simulink model "SYSTEMCOMPLEX"  (R2025b)
settings: Solver=VariableStepAuto  StartTime=0.0  StopTime=10.0  RelTol=1e-3
(part 2 of 2)

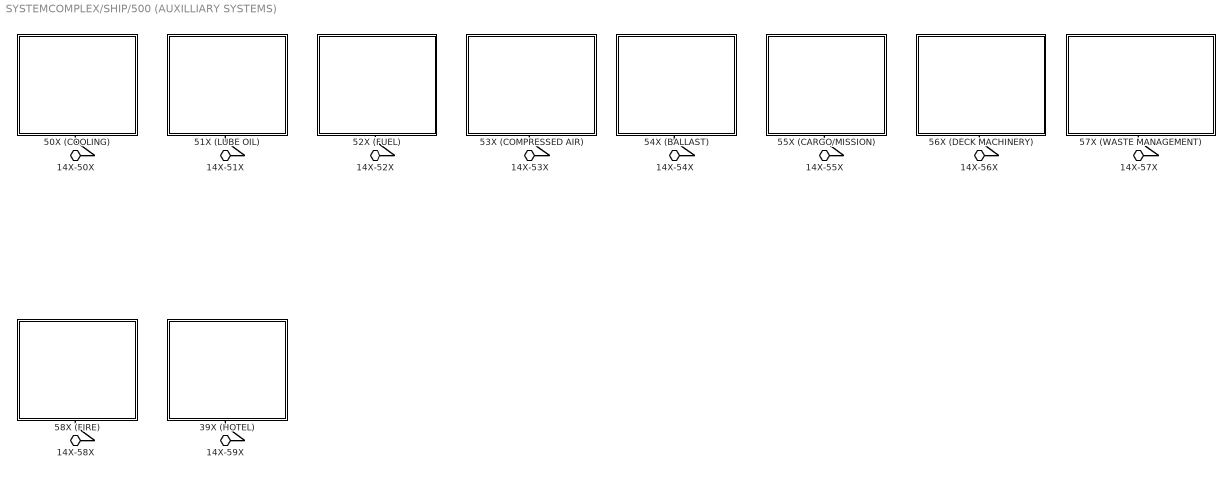
== system SYSTEMCOMPLEX/SHIP/500 (AUXILLIARY SYSTEMS) ==
  39X (HOTEL) : Subsystem
      settings: PortSchema="{\"entries\":[{\"content\":{\"headerSize\":26,\"margin\":15,\"minimumSpacing\":25,\"sides\":[{\"content\":{},\"type\":\"ConnectorPlacement.EquallySpacedRectSide\",\"uuid\":\"c62bca68-e99b-4d4a-8c3b-c9a3c6520291\"},{\"content\":{\"side\":\"RIGHT\"},\"type\":\"ConnectorPlacement.EquallySpacedRectSide\",\"uuid\":\"9f78cd75-5645-4950-8d66-9f0d33627f1f\"},{\"content\":{\"side\":\"TOP\"},\"type\":\"ConnectorPlacement.EquallySpacedRectSide\",\"uuid\":\"f95077c9-4a6b-4bf1-8b13-59697d659817\"},{\"content\":{\"connectorIds\":[\"RConn1\"],\"side\":\"BOTTOM\"},\"type\":\"ConnectorPlacement.EquallySpacedRectSide\",\"uuid\":\"0006d70a-f92f-457d-a614-8f3c10052d85\"}]},\"type\":\"ConnectorPlacement.EquallySpacedConnector\",\"uuid\":\"da1ef182-4ed3-4fb4-823f-e8eb0a5ecd15\"}],\"packageUris\":[\"http://schema.mathworks.com/mf0/Connector/R2020b\"],\"version\":\"1.0\"}"
  50X (COOLING) : Subsystem
      settings: PortSchema="{\"entries\":[{\"content\":{\"headerSize\":26,\"margin\":15,\"minimumSpacing\":25,\"sides\":[{\"content\":{},\"type\":\"ConnectorPlacement.EquallySpacedRectSide\",\"uuid\":\"c62bca68-e99b-4d4a-8c3b-c9a3c6520291\"},{\"content\":{\"side\":\"RIGHT\"},\"type\":\"ConnectorPlacement.EquallySpacedRectSide\",\"uuid\":\"9f78cd75-5645-4950-8d66-9f0d33627f1f\"},{\"content\":{\"side\":\"TOP\"},\"type\":\"ConnectorPlacement.EquallySpacedRectSide\",\"uuid\":\"f95077c9-4a6b-4bf1-8b13-59697d659817\"},{\"content\":{\"connectorIds\":[\"RConn1\"],\"side\":\"BOTTOM\"},\"type\":\"ConnectorPlacement.EquallySpacedRectSide\",\"uuid\":\"c6240b2d-810b-4c18-b4a4-281a824149ba\"}]},\"type\":\"ConnectorPlacement.EquallySpacedConnector\",\"uuid\":\"da1ef182-4ed3-4fb4-823f-e8eb0a5ecd15\"}],\"packageUris\":[\"http://schema.mathworks.com/mf0/Connector/R2020b\"],\"version\":\"1.0\"}"
  51X (LUBE OIL) : Subsystem
      settings: PortSchema="{\"entries\":[{\"content\":{\"headerSize\":26,\"margin\":15,\"minimumSpacing\":25,\"sides\":[{\"content\":{},\"type\":\"ConnectorPlacement.EquallySpacedRectSide\",\"uuid\":\"c62bca68-e99b-4d4a-8c3b-c9a3c6520291\"},{\"content\":{\"side\":\"RIGHT\"},\"type\":\"ConnectorPlacement.EquallySpacedRectSide\",\"uuid\":\"9f78cd75-5645-4950-8d66-9f0d33627f1f\"},{\"content\":{\"side\":\"TOP\"},\"type\":\"ConnectorPlacement.EquallySpacedRectSide\",\"uuid\":\"f95077c9-4a6b-4bf1-8b13-59697d659817\"},{\"content\":{\"connectorIds\":[\"RConn1\"],\"side\":\"BOTTOM\"},\"type\":\"ConnectorPlacement.EquallySpacedRectSide\",\"uuid\":\"3fff4ade-ce74-4018-83c1-67b82f153eaa\"}]},\"type\":\"ConnectorPlacement.EquallySpacedConnector\",\"uuid\":\"da1ef182-4ed3-4fb4-823f-e8eb0a5ecd15\"}],\"packageUris\":[\"http://schema.mathworks.com/mf0/Connector/R2020b\"],\"version\":\"1.0\"}"
  52X (FUEL) : Subsystem
      settings: PortSchema="{\"entries\":[{\"content\":{\"headerSize\":26,\"margin\":15,\"minimumSpacing\":25,\"sides\":[{\"content\":{},\"type\":\"ConnectorPlacement.EquallySpacedRectSide\",\"uuid\":\"c62bca68-e99b-4d4a-8c3b-c9a3c6520291\"},{\"content\":{\"side\":\"RIGHT\"},\"type\":\"ConnectorPlacement.EquallySpacedRectSide\",\"uuid\":\"9f78cd75-5645-4950-8d66-9f0d33627f1f\"},{\"content\":{\"side\":\"TOP\"},\"type\":\"ConnectorPlacement.EquallySpacedRectSide\",\"uuid\":\"f95077c9-4a6b-4bf1-8b13-59697d659817\"},{\"content\":{\"connectorIds\":[\"RConn1\"],\"side\":\"BOTTOM\"},\"type\":\"ConnectorPlacement.EquallySpacedRectSide\",\"uuid\":\"83459f23-a1ce-4fbc-97a5-e0f72e97561e\"}]},\"type\":\"ConnectorPlacement.EquallySpacedConnector\",\"uuid\":\"da1ef182-4ed3-4fb4-823f-e8eb0a5ecd15\"}],\"packageUris\":[\"http://schema.mathworks.com/mf0/Connector/R2020b\"],\"version\":\"1.0\"}"
  53X (COMPRESSED AIR) : Subsystem
      settings: PortSchema="{\"entries\":[{\"content\":{\"headerSize\":26,\"margin\":15,\"minimumSpacing\":25,\"sides\":[{\"content\":{},\"type\":\"ConnectorPlacement.EquallySpacedRectSide\",\"uuid\":\"c62bca68-e99b-4d4a-8c3b-c9a3c6520291\"},{\"content\":{\"side\":\"RIGHT\"},\"type\":\"ConnectorPlacement.EquallySpacedRectSide\",\"uuid\":\"9f78cd75-5645-4950-8d66-9f0d33627f1f\"},{\"content\":{\"side\":\"TOP\"},\"type\":\"ConnectorPlacement.EquallySpacedRectSide\",\"uuid\":\"f95077c9-4a6b-4bf1-8b13-59697d659817\"},{\"content\":{\"connectorIds\":[\"RConn1\"],\"side\":\"BOTTOM\"},\"type\":\"ConnectorPlacement.EquallySpacedRectSide\",\"uuid\":\"74713995-6afe-49df-9f00-ac1603891ac3\"}]},\"type\":\"ConnectorPlacement.EquallySpacedConnector\",\"uuid\":\"da1ef182-4ed3-4fb4-823f-e8eb0a5ecd15\"}],\"packageUris\":[\"http://schema.mathworks.com/mf0/Connector/R2020b\"],\"version\":\"1.0\"}"
  54X (BALLAST) : Subsystem
      settings: PortSchema="{\"entries\":[{\"content\":{\"headerSize\":26,\"margin\":15,\"minimumSpacing\":25,\"sides\":[{\"content\":{},\"type\":\"ConnectorPlacement.EquallySpacedRectSide\",\"uuid\":\"c62bca68-e99b-4d4a-8c3b-c9a3c6520291\"},{\"content\":{\"side\":\"RIGHT\"},\"type\":\"ConnectorPlacement.EquallySpacedRectSide\",\"uuid\":\"9f78cd75-5645-4950-8d66-9f0d33627f1f\"},{\"content\":{\"side\":\"TOP\"},\"type\":\"ConnectorPlacement.EquallySpacedRectSide\",\"uuid\":\"f95077c9-4a6b-4bf1-8b13-59697d659817\"},{\"content\":{\"connectorIds\":[\"RConn1\"],\"side\":\"BOTTOM\"},\"type\":\"ConnectorPlacement.EquallySpacedRectSide\",\"uuid\":\"68d91af7-5bf5-42be-a1d8-d4884acaee75\"}]},\"type\":\"ConnectorPlacement.EquallySpacedConnector\",\"uuid\":\"da1ef182-4ed3-4fb4-823f-e8eb0a5ecd15\"}],\"packageUris\":[\"http://schema.mathworks.com/mf0/Connector/R2020b\"],\"version\":\"1.0\"}"
  55X (CARGO/MISSION) : Subsystem
      settings: PortSchema="{\"entries\":[{\"content\":{\"headerSize\":26,\"margin\":15,\"minimumSpacing\":25,\"sides\":[{\"content\":{},\"type\":\"ConnectorPlacement.EquallySpacedRectSide\",\"uuid\":\"c62bca68-e99b-4d4a-8c3b-c9a3c6520291\"},{\"content\":{\"side\":\"RIGHT\"},\"type\":\"ConnectorPlacement.EquallySpacedRectSide\",\"uuid\":\"9f78cd75-5645-4950-8d66-9f0d33627f1f\"},{\"content\":{\"side\":\"TOP\"},\"type\":\"ConnectorPlacement.EquallySpacedRectSide\",\"uuid\":\"f95077c9-4a6b-4bf1-8b13-59697d659817\"},{\"content\":{\"connectorIds\":[\"RConn1\"],\"side\":\"BOTTOM\"},\"type\":\"ConnectorPlacement.EquallySpacedRectSide\",\"uuid\":\"082ae5ab-4f38-4cbc-8d3b-78d157006bcc\"}]},\"type\":\"ConnectorPlacement.EquallySpacedConnector\",\"uuid\":\"da1ef182-4ed3-4fb4-823f-e8eb0a5ecd15\"}],\"packageUris\":[\"http://schema.mathworks.com/mf0/Connector/R2020b\"],\"version\":\"1.0\"}"
  56X (DECK MACHINERY) : Subsystem
      settings: PortSchema="{\"entries\":[{\"content\":{\"headerSize\":26,\"margin\":15,\"minimumSpacing\":25,\"sides\":[{\"content\":{},\"type\":\"ConnectorPlacement.EquallySpacedRectSide\",\"uuid\":\"c62bca68-e99b-4d4a-8c3b-c9a3c6520291\"},{\"content\":{\"side\":\"RIGHT\"},\"type\":\"ConnectorPlacement.EquallySpacedRectSide\",\"uuid\":\"9f78cd75-5645-4950-8d66-9f0d33627f1f\"},{\"content\":{\"side\":\"TOP\"},\"type\":\"ConnectorPlacement.EquallySpacedRectSide\",\"uuid\":\"f95077c9-4a6b-4bf1-8b13-59697d659817\"},{\"content\":{\"connectorIds\":[\"RConn1\"],\"side\":\"BOTTOM\"},\"type\":\"ConnectorPlacement.EquallySpacedRectSide\",\"uuid\":\"aa3da118-94c8-43a4-9a24-28ea9b935bf4\"}]},\"type\":\"ConnectorPlacement.EquallySpacedConnector\",\"uuid\":\"da1ef182-4ed3-4fb4-823f-e8eb0a5ecd15\"}],\"packageUris\":[\"http://schema.mathworks.com/mf0/Connector/R2020b\"],\"version\":\"1.0\"}"
  57X (WASTE MANAGEMENT) : Subsystem
      settings: PortSchema="{\"entries\":[{\"content\":{\"headerSize\":26,\"margin\":15,\"minimumSpacing\":25,\"sides\":[{\"content\":{},\"type\":\"ConnectorPlacement.EquallySpacedRectSide\",\"uuid\":\"c62bca68-e99b-4d4a-8c3b-c9a3c6520291\"},{\"content\":{\"side\":\"RIGHT\"},\"type\":\"ConnectorPlacement.EquallySpacedRectSide\",\"uuid\":\"9f78cd75-5645-4950-8d66-9f0d33627f1f\"},{\"content\":{\"side\":\"TOP\"},\"type\":\"ConnectorPlacement.EquallySpacedRectSide\",\"uuid\":\"f95077c9-4a6b-4bf1-8b13-59697d659817\"},{\"content\":{\"connectorIds\":[\"RConn1\"],\"side\":\"BOTTOM\"},\"type\":\"ConnectorPlacement.EquallySpacedRectSide\",\"uuid\":\"a20644fe-ab63-4955-9ccf-f975c8687a67\"}]},\"type\":\"ConnectorPlacement.EquallySpacedConnector\",\"uuid\":\"da1ef182-4ed3-4fb4-823f-e8eb0a5ecd15\"}],\"packageUris\":[\"http://schema.mathworks.com/mf0/Connector/R2020b\"],\"version\":\"1.0\"}"
  58X (FIRE) : Subsystem
      settings: PortSchema="{\"entries\":[{\"content\":{\"headerSize\":26,\"margin\":15,\"minimumSpacing\":25,\"sides\":[{\"content\":{},\"type\":\"ConnectorPlacement.EquallySpacedRectSide\",\"uuid\":\"c62bca68-e99b-4d4a-8c3b-c9a3c6520291\"},{\"content\":{\"side\":\"RIGHT\"},\"type\":\"ConnectorPlacement.EquallySpacedRectSide\",\"uuid\":\"9f78cd75-5645-4950-8d66-9f0d33627f1f\"},{\"content\":{\"side\":\"TOP\"},\"type\":\"ConnectorPlacement.EquallySpacedRectSide\",\"uuid\":\"f95077c9-4a6b-4bf1-8b13-59697d659817\"},{\"content\":{\"connectorIds\":[\"RConn1\"],\"side\":\"BOTTOM\"},\"type\":\"ConnectorPlacement.EquallySpacedRectSide\",\"uuid\":\"000ad661-d3a1-4abe-a6ec-7b31413b8243\"}]},\"type\":\"ConnectorPlacement.EquallySpacedConnector\",\"uuid\":\"da1ef182-4ed3-4fb4-823f-e8eb0a5ecd15\"}],\"packageUris\":[\"http://schema.mathworks.com/mf0/Connector/R2020b\"],\"version\":\"1.0\"}"
  14X-50X : PMIOPort  Side=Left
  14X-51X : PMIOPort  Port=2  Side=Left
  14X-52X : PMIOPort  Port=3  Side=Left
  14X-53X : PMIOPort  Port=4  Side=Left
  14X-54X : PMIOPort  Port=5  Side=Left
  14X-55X : PMIOPort  Port=6  Side=Left
  14X-56X : PMIOPort  Port=7  Side=Left
  14X-57X : PMIOPort  Port=8  Side=Left
  14X-58X : PMIOPort  Port=9  Side=Left
  14X-59X : PMIOPort  Port=10  Side=Left
  connections:
  14X-50X/RConn1 -- 50X (COOLING)/RConn1
  14X-51X/RConn1 -- 51X (LUBE OIL)/RConn1
  14X-52X/RConn1 -- 52X (FUEL)/RConn1
  14X-53X/RConn1 -- 53X (COMPRESSED AIR)/RConn1
  14X-54X/RConn1 -- 54X (BALLAST)/RConn1
  14X-55X/RConn1 -- 55X (CARGO/MISSION)/RConn1
  14X-56X/RConn1 -- 56X (DECK MACHINERY)/RConn1
  14X-57X/RConn1 -- 57X (WASTE MANAGEMENT)/RConn1
  14X-58X/RConn1 -- 58X (FIRE)/RConn1
  14X-59X/RConn1 -- 39X (HOTEL)/RConn1

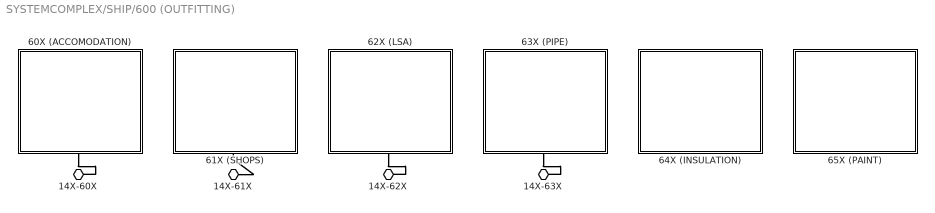
== system SYSTEMCOMPLEX/SHIP/600 (OUTFITTING) ==
  60X (ACCOMODATION) : Subsystem
      settings: PortSchema="{\"entries\":[{\"content\":{\"headerSize\":26,\"margin\":15,\"minimumSpacing\":25,\"sides\":[{\"content\":{},\"type\":\"ConnectorPlacement.EquallySpacedRectSide\",\"uuid\":\"c62bca68-e99b-4d4a-8c3b-c9a3c6520291\"},{\"content\":{\"side\":\"RIGHT\"},\"type\":\"ConnectorPlacement.EquallySpacedRectSide\",\"uuid\":\"9f78cd75-5645-4950-8d66-9f0d33627f1f\"},{\"content\":{\"side\":\"TOP\"},\"type\":\"ConnectorPlacement.EquallySpacedRectSide\",\"uuid\":\"f95077c9-4a6b-4bf1-8b13-59697d659817\"},{\"content\":{\"connectorIds\":[\"RConn1\"],\"side\":\"BOTTOM\"},\"type\":\"ConnectorPlacement.EquallySpacedRectSide\",\"uuid\":\"e1b75886-8c6a-41df-87a3-90c3eee2745e\"}]},\"type\":\"ConnectorPlacement.EquallySpacedConnector\",\"uuid\":\"da1ef182-4ed3-4fb4-823f-e8eb0a5ecd15\"}],\"packageUris\":[\"http://schema.mathworks.com/mf0/Connector/R2020b\"],\"version\":\"1.0\"}"
  61X (SHOPS) : Subsystem
      settings: PortSchema="{\"entries\":[{\"content\":{\"headerSize\":26,\"margin\":15,\"minimumSpacing\":25,\"sides\":[{\"content\":{},\"type\":\"ConnectorPlacement.EquallySpacedRectSide\",\"uuid\":\"c62bca68-e99b-4d4a-8c3b-c9a3c6520291\"},{\"content\":{\"side\":\"RIGHT\"},\"type\":\"ConnectorPlacement.EquallySpacedRectSide\",\"uuid\":\"9f78cd75-5645-4950-8d66-9f0d33627f1f\"},{\"content\":{\"side\":\"TOP\"},\"type\":\"ConnectorPlacement.EquallySpacedRectSide\",\"uuid\":\"f95077c9-4a6b-4bf1-8b13-59697d659817\"},{\"content\":{\"connectorIds\":[\"RConn1\"],\"side\":\"BOTTOM\"},\"type\":\"ConnectorPlacement.EquallySpacedRectSide\",\"uuid\":\"eda74852-aada-4e88-83db-568f63a98b4f\"}]},\"type\":\"ConnectorPlacement.EquallySpacedConnector\",\"uuid\":\"da1ef182-4ed3-4fb4-823f-e8eb0a5ecd15\"}],\"packageUris\":[\"http://schema.mathworks.com/mf0/Connector/R2020b\"],\"version\":\"1.0\"}"
  62X (LSA) : Subsystem
      settings: PortSchema="{\"entries\":[{\"content\":{\"headerSize\":26,\"margin\":15,\"minimumSpacing\":25,\"sides\":[{\"content\":{},\"type\":\"ConnectorPlacement.EquallySpacedRectSide\",\"uuid\":\"c62bca68-e99b-4d4a-8c3b-c9a3c6520291\"},{\"content\":{\"side\":\"RIGHT\"},\"type\":\"ConnectorPlacement.EquallySpacedRectSide\",\"uuid\":\"9f78cd75-5645-4950-8d66-9f0d33627f1f\"},{\"content\":{\"side\":\"TOP\"},\"type\":\"ConnectorPlacement.EquallySpacedRectSide\",\"uuid\":\"f95077c9-4a6b-4bf1-8b13-59697d659817\"},{\"content\":{\"connectorIds\":[\"RConn1\"],\"side\":\"BOTTOM\"},\"type\":\"ConnectorPlacement.EquallySpacedRectSide\",\"uuid\":\"eb68c783-c2b7-425c-a30e-1e7ae8b8046b\"}]},\"type\":\"ConnectorPlacement.EquallySpacedConnector\",\"uuid\":\"da1ef182-4ed3-4fb4-823f-e8eb0a5ecd15\"}],\"packageUris\":[\"http://schema.mathworks.com/mf0/Connector/R2020b\"],\"version\":\"1.0\"}"
  63X (PIPE) : Subsystem
      settings: PortSchema="{\"entries\":[{\"content\":{\"headerSize\":26,\"margin\":15,\"minimumSpacing\":25,\"sides\":[{\"content\":{},\"type\":\"ConnectorPlacement.EquallySpacedRectSide\",\"uuid\":\"c62bca68-e99b-4d4a-8c3b-c9a3c6520291\"},{\"content\":{\"side\":\"RIGHT\"},\"type\":\"ConnectorPlacement.EquallySpacedRectSide\",\"uuid\":\"9f78cd75-5645-4950-8d66-9f0d33627f1f\"},{\"content\":{\"side\":\"TOP\"},\"type\":\"ConnectorPlacement.EquallySpacedRectSide\",\"uuid\":\"f95077c9-4a6b-4bf1-8b13-59697d659817\"},{\"content\":{\"connectorIds\":[\"RConn1\"],\"side\":\"BOTTOM\"},\"type\":\"ConnectorPlacement.EquallySpacedRectSide\",\"uuid\":\"9d615349-c26c-46cb-ae8c-7a410c7bc294\"}]},\"type\":\"ConnectorPlacement.EquallySpacedConnector\",\"uuid\":\"da1ef182-4ed3-4fb4-823f-e8eb0a5ecd15\"}],\"packageUris\":[\"http://schema.mathworks.com/mf0/Connector/R2020b\"],\"version\":\"1.0\"}"
  64X (INSULATION) : Subsystem
      settings: PortSchema="{\"entries\":[{\"content\":{\"headerSize\":26,\"margin\":15,\"minimumSpacing\":25,\"sides\":[{\"content\":{},\"type\":\"ConnectorPlacement.EquallySpacedRectSide\",\"uuid\":\"c62bca68-e99b-4d4a-8c3b-c9a3c6520291\"},{\"content\":{\"side\":\"RIGHT\"},\"type\":\"ConnectorPlacement.EquallySpacedRectSide\",\"uuid\":\"9f78cd75-5645-4950-8d66-9f0d33627f1f\"},{\"content\":{\"side\":\"TOP\"},\"type\":\"ConnectorPlacement.EquallySpacedRectSide\",\"uuid\":\"f95077c9-4a6b-4bf1-8b13-59697d659817\"},{\"content\":{\"side\":\"BOTTOM\"},\"type\":\"ConnectorPlacement.EquallySpacedRectSide\",\"uuid\":\"a124c561-1965-4589-a1a5-91c1941cde96\"}]},\"type\":\"ConnectorPlacement.EquallySpacedConnector\",\"uuid\":\"da1ef182-4ed3-4fb4-823f-e8eb0a5ecd15\"}],\"packageUris\":[\"http://schema.mathworks.com/mf0/Connector/R2020b\"],\"version\":\"1.0\"}"
  65X (PAINT) : Subsystem
      settings: PortSchema="{\"entries\":[{\"content\":{\"headerSize\":26,\"margin\":15,\"minimumSpacing\":25,\"sides\":[{\"content\":{},\"type\":\"ConnectorPlacement.EquallySpacedRectSide\",\"uuid\":\"c62bca68-e99b-4d4a-8c3b-c9a3c6520291\"},{\"content\":{\"side\":\"RIGHT\"},\"type\":\"ConnectorPlacement.EquallySpacedRectSide\",\"uuid\":\"9f78cd75-5645-4950-8d66-9f0d33627f1f\"},{\"content\":{\"side\":\"TOP\"},\"type\":\"ConnectorPlacement.EquallySpacedRectSide\",\"uuid\":\"f95077c9-4a6b-4bf1-8b13-59697d659817\"},{\"content\":{\"side\":\"BOTTOM\"},\"type\":\"ConnectorPlacement.EquallySpacedRectSide\",\"uuid\":\"a1cd9f97-e758-4f5e-aae1-f061bacce1d6\"}]},\"type\":\"ConnectorPlacement.EquallySpacedConnector\",\"uuid\":\"da1ef182-4ed3-4fb4-823f-e8eb0a5ecd15\"}],\"packageUris\":[\"http://schema.mathworks.com/mf0/Connector/R2020b\"],\"version\":\"1.0\"}"
  14X-60X : PMIOPort  Side=Left
  14X-61X : PMIOPort  Port=2  Side=Left
  14X-62X : PMIOPort  Port=3  Side=Left
  14X-63X : PMIOPort  Port=4  Side=Left
  connections:
  60X (ACCOMODATION)/RConn1 -- 14X-60X/RConn1
  14X-61X/RConn1 -- 61X (SHOPS)/RConn1
  62X (LSA)/RConn1 -- 14X-62X/RConn1
  63X (PIPE)/RConn1 -- 14X-63X/RConn1

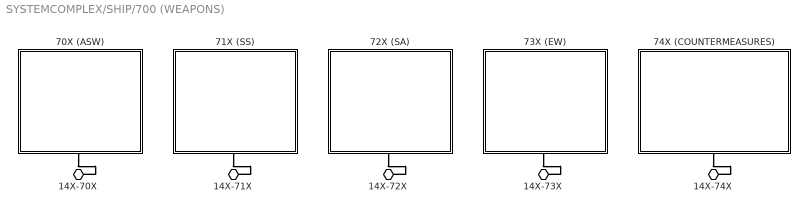
== system SYSTEMCOMPLEX/SHIP/700 (WEAPONS) ==
  70X (ASW) : Subsystem
      settings: PortSchema="{\"entries\":[{\"content\":{\"headerSize\":26,\"margin\":15,\"minimumSpacing\":25,\"sides\":[{\"content\":{},\"type\":\"ConnectorPlacement.EquallySpacedRectSide\",\"uuid\":\"c62bca68-e99b-4d4a-8c3b-c9a3c6520291\"},{\"content\":{\"side\":\"RIGHT\"},\"type\":\"ConnectorPlacement.EquallySpacedRectSide\",\"uuid\":\"9f78cd75-5645-4950-8d66-9f0d33627f1f\"},{\"content\":{\"side\":\"TOP\"},\"type\":\"ConnectorPlacement.EquallySpacedRectSide\",\"uuid\":\"f95077c9-4a6b-4bf1-8b13-59697d659817\"},{\"content\":{\"connectorIds\":[\"RConn1\"],\"side\":\"BOTTOM\"},\"type\":\"ConnectorPlacement.EquallySpacedRectSide\",\"uuid\":\"8c7f8e96-6909-4916-93d9-769c06356a06\"}]},\"type\":\"ConnectorPlacement.EquallySpacedConnector\",\"uuid\":\"da1ef182-4ed3-4fb4-823f-e8eb0a5ecd15\"}],\"packageUris\":[\"http://schema.mathworks.com/mf0/Connector/R2020b\"],\"version\":\"1.0\"}"
  71X (SS) : Subsystem
      settings: PortSchema="{\"entries\":[{\"content\":{\"headerSize\":26,\"margin\":15,\"minimumSpacing\":25,\"sides\":[{\"content\":{},\"type\":\"ConnectorPlacement.EquallySpacedRectSide\",\"uuid\":\"c62bca68-e99b-4d4a-8c3b-c9a3c6520291\"},{\"content\":{\"side\":\"RIGHT\"},\"type\":\"ConnectorPlacement.EquallySpacedRectSide\",\"uuid\":\"9f78cd75-5645-4950-8d66-9f0d33627f1f\"},{\"content\":{\"side\":\"TOP\"},\"type\":\"ConnectorPlacement.EquallySpacedRectSide\",\"uuid\":\"f95077c9-4a6b-4bf1-8b13-59697d659817\"},{\"content\":{\"connectorIds\":[\"RConn1\"],\"side\":\"BOTTOM\"},\"type\":\"ConnectorPlacement.EquallySpacedRectSide\",\"uuid\":\"b7e9c118-18c2-4f79-8577-1bc6c54a25a2\"}]},\"type\":\"ConnectorPlacement.EquallySpacedConnector\",\"uuid\":\"da1ef182-4ed3-4fb4-823f-e8eb0a5ecd15\"}],\"packageUris\":[\"http://schema.mathworks.com/mf0/Connector/R2020b\"],\"version\":\"1.0\"}"
  72X (SA) : Subsystem
      settings: PortSchema="{\"entries\":[{\"content\":{\"headerSize\":26,\"margin\":15,\"minimumSpacing\":25,\"sides\":[{\"content\":{},\"type\":\"ConnectorPlacement.EquallySpacedRectSide\",\"uuid\":\"c62bca68-e99b-4d4a-8c3b-c9a3c6520291\"},{\"content\":{\"side\":\"RIGHT\"},\"type\":\"ConnectorPlacement.EquallySpacedRectSide\",\"uuid\":\"9f78cd75-5645-4950-8d66-9f0d33627f1f\"},{\"content\":{\"side\":\"TOP\"},\"type\":\"ConnectorPlacement.EquallySpacedRectSide\",\"uuid\":\"f95077c9-4a6b-4bf1-8b13-59697d659817\"},{\"content\":{\"connectorIds\":[\"RConn1\"],\"side\":\"BOTTOM\"},\"type\":\"ConnectorPlacement.EquallySpacedRectSide\",\"uuid\":\"987dd861-726c-4128-8a91-eb8cbbfb100b\"}]},\"type\":\"ConnectorPlacement.EquallySpacedConnector\",\"uuid\":\"da1ef182-4ed3-4fb4-823f-e8eb0a5ecd15\"}],\"packageUris\":[\"http://schema.mathworks.com/mf0/Connector/R2020b\"],\"version\":\"1.0\"}"
  73X (EW) : Subsystem
      settings: PortSchema="{\"entries\":[{\"content\":{\"headerSize\":26,\"margin\":15,\"minimumSpacing\":25,\"sides\":[{\"content\":{},\"type\":\"ConnectorPlacement.EquallySpacedRectSide\",\"uuid\":\"c62bca68-e99b-4d4a-8c3b-c9a3c6520291\"},{\"content\":{\"side\":\"RIGHT\"},\"type\":\"ConnectorPlacement.EquallySpacedRectSide\",\"uuid\":\"9f78cd75-5645-4950-8d66-9f0d33627f1f\"},{\"content\":{\"side\":\"TOP\"},\"type\":\"ConnectorPlacement.EquallySpacedRectSide\",\"uuid\":\"f95077c9-4a6b-4bf1-8b13-59697d659817\"},{\"content\":{\"connectorIds\":[\"RConn1\"],\"side\":\"BOTTOM\"},\"type\":\"ConnectorPlacement.EquallySpacedRectSide\",\"uuid\":\"ab95cec6-1633-4770-81aa-00d322a1e6a9\"}]},\"type\":\"ConnectorPlacement.EquallySpacedConnector\",\"uuid\":\"da1ef182-4ed3-4fb4-823f-e8eb0a5ecd15\"}],\"packageUris\":[\"http://schema.mathworks.com/mf0/Connector/R2020b\"],\"version\":\"1.0\"}"
  74X (COUNTERMEASURES) : Subsystem
      settings: PortSchema="{\"entries\":[{\"content\":{\"headerSize\":26,\"margin\":15,\"minimumSpacing\":25,\"sides\":[{\"content\":{},\"type\":\"ConnectorPlacement.EquallySpacedRectSide\",\"uuid\":\"c62bca68-e99b-4d4a-8c3b-c9a3c6520291\"},{\"content\":{\"side\":\"RIGHT\"},\"type\":\"ConnectorPlacement.EquallySpacedRectSide\",\"uuid\":\"9f78cd75-5645-4950-8d66-9f0d33627f1f\"},{\"content\":{\"side\":\"TOP\"},\"type\":\"ConnectorPlacement.EquallySpacedRectSide\",\"uuid\":\"f95077c9-4a6b-4bf1-8b13-59697d659817\"},{\"content\":{\"connectorIds\":[\"RConn1\"],\"side\":\"BOTTOM\"},\"type\":\"ConnectorPlacement.EquallySpacedRectSide\",\"uuid\":\"d305fc0d-b8d9-47aa-9958-864ada4c8608\"}]},\"type\":\"ConnectorPlacement.EquallySpacedConnector\",\"uuid\":\"da1ef182-4ed3-4fb4-823f-e8eb0a5ecd15\"}],\"packageUris\":[\"http://schema.mathworks.com/mf0/Connector/R2020b\"],\"version\":\"1.0\"}"
  14X-70X : PMIOPort  Side=Left
  14X-71X : PMIOPort  Port=2  Side=Left
  14X-72X : PMIOPort  Port=3  Side=Left
  14X-73X : PMIOPort  Port=4  Side=Left
  14X-74X : PMIOPort  Port=5  Side=Left
  connections:
  70X (ASW)/RConn1 -- 14X-70X/RConn1
  71X (SS)/RConn1 -- 14X-71X/RConn1
  72X (SA)/RConn1 -- 14X-72X/RConn1
  73X (EW)/RConn1 -- 14X-73X/RConn1
  74X (COUNTERMEASURES)/RConn1 -- 14X-74X/RConn1

== system SYSTEMCOMPLEX/SHIP/100 (HULL)/10X (PLATE) ==
  14X-10X : PMIOPort  Side=Right

== system SYSTEMCOMPLEX/SHIP/100 (HULL)/11X (FRAMING) ==
  14X-11X : PMIOPort  Side=Right

== system SYSTEMCOMPLEX/SHIP/100 (HULL)/12X (GIRDERS) ==
  14X-12X : PMIOPort  Side=Right

== system SYSTEMCOMPLEX/SHIP/100 (HULL)/13X (STIFFENERS) ==
  14X-13X : PMIOPort  Side=Right

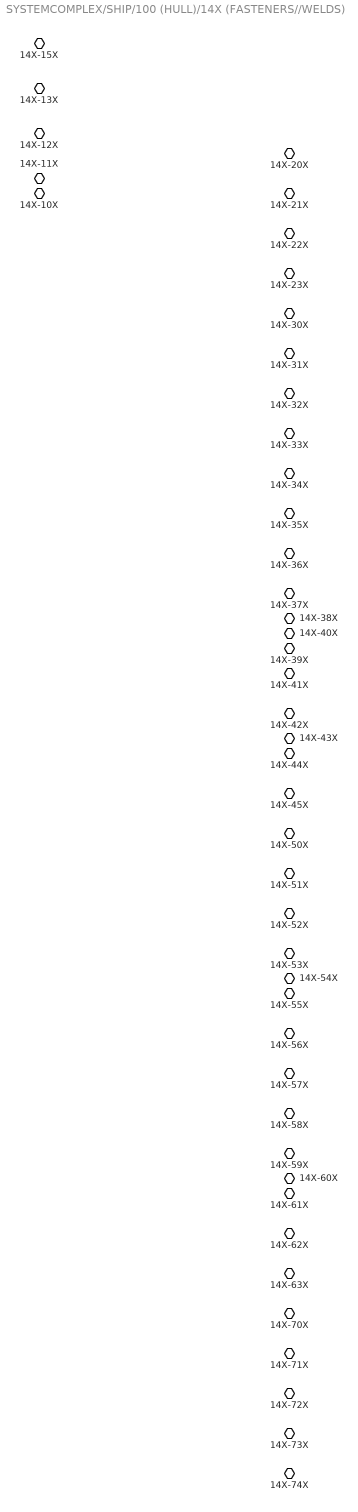
== system SYSTEMCOMPLEX/SHIP/100 (HULL)/14X (FASTENERS//WELDS) ==
  14X-15X : PMIOPort  Side=Left
  14X-13X : PMIOPort  Port=2  Side=Left
  14X-12X : PMIOPort  Port=3  Side=Left
  14X-11X : PMIOPort  Port=4  Side=Left
  14X-10X : PMIOPort  Port=5  Side=Left
  14X-20X : PMIOPort  Port=6  Side=Right
  14X-21X : PMIOPort  Port=7  Side=Right
  14X-22X : PMIOPort  Port=8  Side=Right
  14X-23X : PMIOPort  Port=9  Side=Right
  14X-30X : PMIOPort  Port=10  Side=Right
  14X-31X : PMIOPort  Port=11  Side=Right
  14X-32X : PMIOPort  Port=12  Side=Right
  14X-33X : PMIOPort  Port=13  Side=Right
  14X-34X : PMIOPort  Port=14  Side=Right
  14X-35X : PMIOPort  Port=15  Side=Right
  14X-36X : PMIOPort  Port=16  Side=Right
  14X-37X : PMIOPort  Port=17  Side=Right
  14X-38X : PMIOPort  Port=18  Side=Right
  14X-39X : PMIOPort  Port=19  Side=Right
  14X-40X : PMIOPort  Port=20  Side=Right
  14X-41X : PMIOPort  Port=21  Side=Right
  14X-42X : PMIOPort  Port=22  Side=Right
  14X-43X : PMIOPort  Port=23  Side=Right
  14X-44X : PMIOPort  Port=24  Side=Right
  14X-45X : PMIOPort  Port=25  Side=Right
  14X-50X : PMIOPort  Port=26  Side=Right
  14X-51X : PMIOPort  Port=27  Side=Right
  14X-52X : PMIOPort  Port=28  Side=Right
  14X-53X : PMIOPort  Port=29  Side=Right
  14X-54X : PMIOPort  Port=30  Side=Right
  14X-55X : PMIOPort  Port=31  Side=Right
  14X-56X : PMIOPort  Port=32  Side=Right
  14X-57X : PMIOPort  Port=33  Side=Right
  14X-58X : PMIOPort  Port=34  Side=Right
  14X-59X : PMIOPort  Port=35  Side=Right
  14X-60X : PMIOPort  Port=36  Side=Right
  14X-61X : PMIOPort  Port=37  Side=Right
  14X-62X : PMIOPort  Port=38  Side=Right
  14X-63X : PMIOPort  Port=39  Side=Right
  14X-70X : PMIOPort  Port=40  Side=Right
  14X-71X : PMIOPort  Port=41  Side=Right
  14X-72X : PMIOPort  Port=42  Side=Right
  14X-73X : PMIOPort  Port=43  Side=Right
  14X-74X : PMIOPort  Port=44  Side=Right

== system SYSTEMCOMPLEX/SHIP/100 (HULL)/15X (MOUNTINGS) ==
  14X-15X : PMIOPort  Side=Right

== system SYSTEMCOMPLEX/SHIP/200 (PROPULSION)/20X (MAIN ENGINE) ==
  14X-20X : PMIOPort  Side=Left
  TO 23X : PMIOPort  Port=2  Side=Left

== system SYSTEMCOMPLEX/SHIP/200 (PROPULSION)/21X (PROPULSORS) ==
  14X-21X : PMIOPort  Side=Right
  FROM 22X : PMIOPort  Port=2  Side=Right

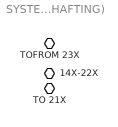
== system SYSTEMCOMPLEX/SHIP/200 (PROPULSION)/22X (SHAFTING) ==
  TOFROM 23X : PMIOPort  Side=Right
  14X-22X : PMIOPort  Port=2  Side=Right
  TO 21X : PMIOPort  Port=3  Side=Right

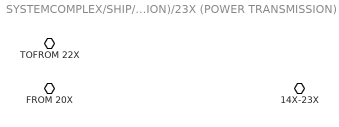
== system SYSTEMCOMPLEX/SHIP/200 (PROPULSION)/23X (POWER TRANSMISSION) ==
  TOFROM 22X : PMIOPort  Side=Left
  FROM 20X : PMIOPort  Port=2  Side=Left
  14X-23X : PMIOPort  Port=3  Side=Right

== system SYSTEMCOMPLEX/SHIP/300 (ELECTRICAL)/30X (LVGS) ==
  14X-30X : PMIOPort  Side=Right

== system SYSTEMCOMPLEX/SHIP/300 (ELECTRICAL)/31X (HVGS) ==
  14X-31X : PMIOPort  Side=Right

== system SYSTEMCOMPLEX/SHIP/300 (ELECTRICAL)/32X (EMER. GS) ==
  14X-32X : PMIOPort  Side=Right

== system SYSTEMCOMPLEX/SHIP/300 (ELECTRICAL)/33X (LVSB) ==
  14X-33X : PMIOPort  Side=Right

== system SYSTEMCOMPLEX/SHIP/300 (ELECTRICAL)/34X (HVSB) ==
  14X-34X : PMIOPort  Side=Right

== system SYSTEMCOMPLEX/SHIP/300 (ELECTRICAL)/35X (TRANSFORMERS) ==
  14X-35X : PMIOPort  Side=Right

== system SYSTEMCOMPLEX/SHIP/300 (ELECTRICAL)/36X (SHORE POWER) ==
  14X-36X : PMIOPort  Side=Right

== system SYSTEMCOMPLEX/SHIP/300 (ELECTRICAL)/37X (BATTERY) ==
  14X-37X : PMIOPort  Side=Right

== system SYSTEMCOMPLEX/SHIP/300 (ELECTRICAL)/38X (FEEDER PANELS) ==
  14X-38X : PMIOPort  Side=Right

== system SYSTEMCOMPLEX/SHIP/300 (ELECTRICAL)/39X (CABLE) ==
  14X-39X : PMIOPort  Side=Right

== system SYSTEMCOMPLEX/SHIP/400 (COMMAND CONTROL)/40X (NAVIGATION//AIS) ==
  14X-40X : PMIOPort  Side=Right

== system SYSTEMCOMPLEX/SHIP/400 (COMMAND CONTROL)/41X (RADIO//SATCOM) ==
  14X-41X : PMIOPort  Side=Right

== system SYSTEMCOMPLEX/SHIP/400 (COMMAND CONTROL)/42X (CONSOLES) ==
  14X-42X : PMIOPort  Side=Right

== system SYSTEMCOMPLEX/SHIP/400 (COMMAND CONTROL)/43X (STEERAGE) ==
  14X-43X : PMIOPort  Side=Right

== system SYSTEMCOMPLEX/SHIP/400 (COMMAND CONTROL)/44X (AIR SURVEILLANCE) ==
  14X-44X : PMIOPort  Side=Right

== system SYSTEMCOMPLEX/SHIP/400 (COMMAND CONTROL)/45X (WATER SURVEILLANCE) ==
  14X-45X : PMIOPort  Side=Right

== system SYSTEMCOMPLEX/SHIP/500 (AUXILLIARY SYSTEMS)/39X (HOTEL) ==
  14X-59X : PMIOPort  Side=Right

== system SYSTEMCOMPLEX/SHIP/500 (AUXILLIARY SYSTEMS)/50X (COOLING) ==
  14X-50X : PMIOPort  Side=Right

== system SYSTEMCOMPLEX/SHIP/500 (AUXILLIARY SYSTEMS)/51X (LUBE OIL) ==
  14X-51X : PMIOPort  Side=Right

== system SYSTEMCOMPLEX/SHIP/500 (AUXILLIARY SYSTEMS)/52X (FUEL) ==
  14X-52X : PMIOPort  Side=Right

== system SYSTEMCOMPLEX/SHIP/500 (AUXILLIARY SYSTEMS)/53X (COMPRESSED AIR) ==
  14X-53X : PMIOPort  Side=Right

== system SYSTEMCOMPLEX/SHIP/500 (AUXILLIARY SYSTEMS)/54X (BALLAST) ==
  14X-54X : PMIOPort  Side=Right

== system SYSTEMCOMPLEX/SHIP/500 (AUXILLIARY SYSTEMS)/55X (CARGO//MISSION) ==
  14X-55X : PMIOPort  Side=Right

== system SYSTEMCOMPLEX/SHIP/500 (AUXILLIARY SYSTEMS)/56X (DECK MACHINERY) ==
  14X-56X : PMIOPort  Side=Right

== system SYSTEMCOMPLEX/SHIP/500 (AUXILLIARY SYSTEMS)/57X (WASTE MANAGEMENT) ==
  14X-57X : PMIOPort  Side=Right

== system SYSTEMCOMPLEX/SHIP/500 (AUXILLIARY SYSTEMS)/58X (FIRE) ==
  14X-58X : PMIOPort  Side=Right

== system SYSTEMCOMPLEX/SHIP/600 (OUTFITTING)/60X (ACCOMODATION) ==
  14X-60X : PMIOPort  Side=Right

== system SYSTEMCOMPLEX/SHIP/600 (OUTFITTING)/61X (SHOPS) ==
  14X-61X : PMIOPort  Side=Right

== system SYSTEMCOMPLEX/SHIP/600 (OUTFITTING)/62X (LSA) ==
  14X-62X : PMIOPort  Side=Right

== system SYSTEMCOMPLEX/SHIP/600 (OUTFITTING)/63X (PIPE) ==
  14X-63X : PMIOPort  Side=Right

== system SYSTEMCOMPLEX/SHIP/600 (OUTFITTING)/64X (INSULATION) ==

== system SYSTEMCOMPLEX/SHIP/600 (OUTFITTING)/65X (PAINT) ==

== system SYSTEMCOMPLEX/SHIP/700 (WEAPONS)/70X (ASW) ==
  14X-70X : PMIOPort  Side=Right

== system SYSTEMCOMPLEX/SHIP/700 (WEAPONS)/71X (SS) ==
  14X-71X : PMIOPort  Side=Right

== system SYSTEMCOMPLEX/SHIP/700 (WEAPONS)/72X (SA) ==
  14X-72X : PMIOPort  Side=Right

== system SYSTEMCOMPLEX/SHIP/700 (WEAPONS)/73X (EW) ==
  14X-73X : PMIOPort  Side=Right

== system SYSTEMCOMPLEX/SHIP/700 (WEAPONS)/74X (COUNTERMEASURES) ==
  14X-74X : PMIOPort  Side=Right
